simulink model "bldc_control"  (R2014b)
settings: Solver=ode3  StartTime=0.0  StopTime=tdur  FixedStep=dt  RelTol=1e-3
values from neighbouring files (symbols this model uses):
  CTRL_MODE = 1    [bldc_control_run.m]
  dt = 0.2    [bldc_control_run.m]    (also in bldc_discrete.m = CONST.dt; bldc_discrete_model.m = CONST.dt; bldc_discrete_torque.m = CONST.dt; bldc_speed_discrete.m = CONST.dt)
  i_kd = 0    [bldc_control_run.m]
  i_ki = 1e3    (= 1000)    [bldc_control_run.m]
  i_kp = 10    [bldc_control_run.m]
  i_tgt = 0.15    [bldc_control_run.m]
  J = 978.548e-6    (= 0.000978548)    [bldc_control_run.m]    (also in bldc_discrete.m = CONST.J; bldc_discrete_model.m = CONST.J; bldc_motor.m = CONST.J; bldc_speed.m = CONST.J)
  spd_kd = 0.00    (= 0)    [bldc_control_run.m]    (also in bldc_speed_discrete.m = CONST.spd_kd)
  spd_ki = 0.10    (= 0.1)    [bldc_control_run.m]    (also in bldc_speed_discrete.m = CONST.spd_ki)
  spd_kp = 0.50    (= 0.5)    [bldc_control_run.m]    (also in bldc_speed_discrete.m = CONST.spd_kp)
  theta_m_0 = 0    [bldc_control_run.m]
  thold = 0.5    [bldc_control_run.m]
  trq_kd = 0    [bldc_control_run.m]    (also in bldc_discrete_torque.m = CONST.trq_kd)
  trq_ki = 5e4    (= 50000)    [bldc_control_run.m]    (also in bldc_discrete_torque.m = CONST.trq_ki)
  trq_kp = 1e3    (= 1000)    [bldc_control_run.m]    (also in bldc_discrete_torque.m = CONST.trq_kp)
  trq_tgt = 0.1e-3    (= 0.0001)    [bldc_control_run.m]
  V_tgt = 2.1    [bldc_control_run.m]
  Vmax = 24    [bldc_control_run.m]
  w_m_0 = 0    [bldc_control_run.m]
  w_tgt = rpm2rps(2000)    [bldc_control_run.m]
libraries: simulink x1, tool x1
settings Model: Creator=root  LastModifiedBy=root
settings DebuggingCC: FrameProcessingCompatibilityMsg=error

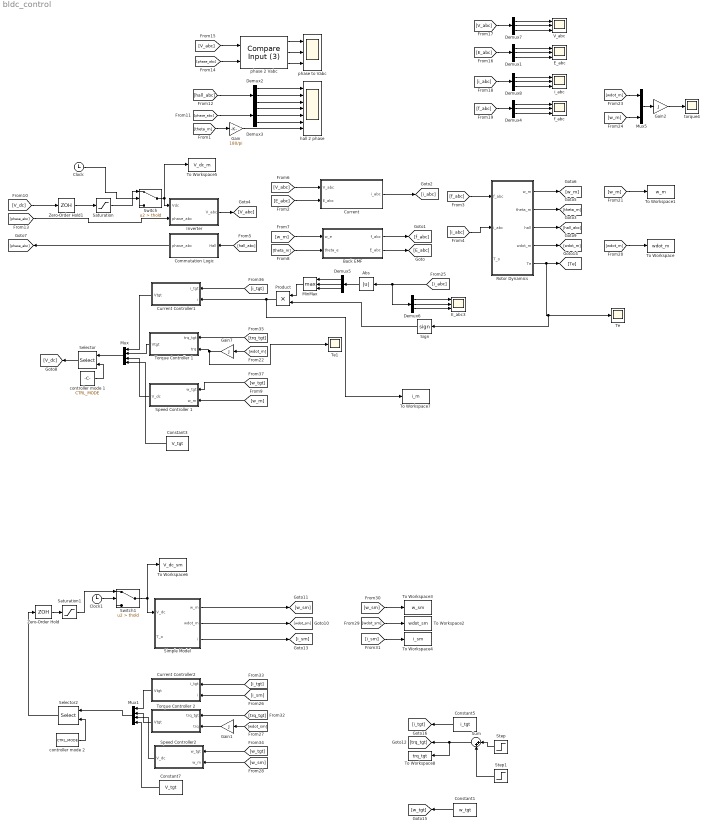
== system bldc_control ==
  Abs : Abs
  Back EMF : Subsystem
  Clock : Clock
  Clock1 : Clock
  Commutation Logic : Subsystem
  Constant1 : Constant  Value=w_tgt
  Constant3 : Constant  Value=V_tgt
  Constant5 : Constant  Value=i_tgt
  Constant7 : Constant  Value=V_tgt
  Current : Subsystem
  Current Controller1 : Subsystem
  Current Controller2 : Subsystem
  Demux{1..8} (8 alike) : Demux  Outputs=3
  E_abc : Scope  NumInputPorts=3
      settings: TimeRange=60  YMin=18000~-5~-5  YMax=20500~5~5  SaveName=ScopeData6
  E_abc3 : Scope  NumInputPorts=3
      settings: TimeRange=5  YMin=-0.05~-0.05~-0.05  YMax=0.05~0.05~0.05  SaveName=ScopeData3
  Gain : Gain  Gain=180/pi
  Gain1 : Gain  Gain=J
  Gain2 : Gain  Gain=J
  Gain7 : Gain  Gain=J
  Inverter : Subsystem
  MinMax : MinMax  Function=max  Inputs=3
  Mux : Mux
  Mux1 : Mux
  Mux5 : Mux  Inputs=3
  Product : Product
  Rotor Dynamics : Subsystem
  Saturation : Saturate  UpperLimit=Vmax  LowerLimit=-Vmax
  Saturation1 : Saturate  UpperLimit=Vmax  LowerLimit=-Vmax
  Selector : Selector  InputPortWidth=4  IndexOptions=Starting index (port)
  Selector2 : Selector  InputPortWidth=4  IndexOptions=Starting index (port)
  Sign : Signum
  Simple Model : Subsystem
  Speed Controller 1 : Subsystem
  Speed Controller2 : Subsystem
  Step : Step  Time=0  After=trq_tgt  SampleTime=0
  Step1 : Step  Time=5  After=-2*trq_tgt  SampleTime=0
  Sum : Sum  Inputs=|++
  Switch : Switch  Criteria=u2 > Threshold  Threshold=thold
  Switch1 : Switch  Criteria=u2 > Threshold  Threshold=thold
  Te : Scope
      settings: TimeRange=1  YMin=1.2e-05  YMax=2.4e-05  SaveName=ScopeData7
  Te1 : Scope
      settings: TimeRange=1  YMin=1.2e-05  YMax=2.4e-05
  To Workspace : ToWorkspace  VariableName=wdot_m  SampleTime=-1
  To Workspace1 : ToWorkspace  VariableName=w_m  SampleTime=-1
  To Workspace2 : ToWorkspace  VariableName=wdot_sm  SampleTime=-1
  To Workspace3 : ToWorkspace  VariableName=w_sm  SampleTime=-1
  To Workspace4 : ToWorkspace  VariableName=i_sm  SampleTime=-1
  To Workspace5 : ToWorkspace  VariableName=V_dc_m  SampleTime=-1
  To Workspace6 : ToWorkspace  VariableName=V_dc_sm  SampleTime=-1
  To Workspace7 : ToWorkspace  VariableName=i_m  SampleTime=-1
  To Workspace8 : ToWorkspace  VariableName=trq_tgt  SampleTime=-1
  Torque Controller 1 : Subsystem
  Torque Controller 2 : Subsystem
  V_abc : Scope  NumInputPorts=3
      settings: TimeRange=60  YMin=18000~-5~-5  YMax=20500~5~5  SaveName=ScopeData5
  Zero-Order Hold : ZeroOrderHold  SampleTime=dt
  Zero-Order Hold1 : ZeroOrderHold  SampleTime=dt
  controller mode 1 : Constant  Value=CTRL_MODE
  controller mode 2 : Constant  Value=CTRL_MODE
  f_abc : Scope  NumInputPorts=3
      settings: TimeRange=60  YMin=18000~-5~-5  YMax=20500~5~5
  hall 2 phase : Scope  NumInputPorts=7
      settings: TimeRange=5  YMin=0~0~0~-1~-1~-1~-200  YMax=1~1~1~1~1~1~200  SaveName=ScopeData8
  i_abc : Scope  NumInputPorts=3
      settings: TimeRange=60  YMin=18000~-5~-5  YMax=20500~5~5  SaveName=ScopeData4
  phase 2 Vabc : tool/Compare Input (3)
  phase to Vabc : Scope  NumInputPorts=3
      settings: TimeRange=5  YMin=-1~-1~-1  YMax=1~1~1  SaveName=ScopeData2
  torque4 : Scope
      settings: TimeRange=1  YMin=1.2e-05  YMax=2.4e-05  SaveName=ScopeData11
  wires:
  [E_abc] -> Current/2(E_abc)
  Back EMF/2(E_abc) -> [E_abc]
  Back EMF/1(f_abc) -> [f_abc]
  [i_abc] -> Rotor Dynamics/2(i_abc)
  Rotor Dynamics/3(hall) -> [hall_abc]
  Commutation Logic/1(phase_abc) -> [phase_abc]
  [V_abc] -> Current/1(V_abc)
  Rotor Dynamics/2(theta_m) -> [theta_m]
  Rotor Dynamics/1(w_m) -> [w_m]
  [theta_m] -> Back EMF/2(theta_e)
  [w_m] -> Back EMF/1(w_e)
  Inverter/1(V_abc) -> [V_abc]
  [hall_abc] -> Commutation Logic/1("Hall ")
  Rotor Dynamics/4(wdot_m) -> [wdot_m]
  Simple Model/1(w_m) -> [w_sm]
  Demux1/3 -> E_abc/3
  Demux1/2 -> E_abc/2
  Demux1/1 -> E_abc/1
  Demux4/3 -> f_abc/3
  Demux4/2 -> f_abc/2
  Demux4/1 -> f_abc/1
  [f_abc] -> Rotor Dynamics/1(f_abc)
  phase 2 Vabc/3 -> phase to Vabc/3
  phase 2 Vabc/2 -> phase to Vabc/2
  phase 2 Vabc/1 -> phase to Vabc/1
  Demux5/1 -> MinMax/1
  Demux5/3 -> MinMax/3
  Demux5/2 -> MinMax/2
  [V_dc] -> Zero-Order Hold1/1
  Current/1(i_abc) -> [i_abc]
  Abs/1 -> Demux5/1
  Simple Model/3(i) -> [i_sm]
  Demux6/3 -> E_abc3/3
  Demux6/2 -> E_abc3/2
  Demux6/1 -> E_abc3/1
  Simple Model/2(wdot_m) -> [wdot_sm]
  Mux5/1 -> Gain2/1
  Constant5/1 -> [i_tgt]
  [i_tgt] -> Current Controller1/1(i_tgt)
  MinMax/1 -> Product/1
  Demux2/3 -> hall 2 phase/3
  Demux2/2 -> hall 2 phase/2
  Demux2/1 -> hall 2 phase/1
  Demux3/2 -> hall 2 phase/5
  Demux3/1 -> hall 2 phase/4
  Demux3/3 -> hall 2 phase/6
  [theta_m] -> Gain/1
  [phase_abc] -> Demux3/1
  Gain/1 -> hall 2 phase/7
  [hall_abc] -> Demux2/1
  [phase_abc] -> Inverter/2(phase_abc)
  [phase_abc] -> phase 2 Vabc/2
  [V_abc] -> phase 2 Vabc/1
  [E_abc] -> Demux1/1
  Demux7/3 -> V_abc/3
  Demux7/2 -> V_abc/2
  Demux7/1 -> V_abc/1
  [V_abc] -> Demux7/1
  Saturation/1 -> Switch/1
  Saturation1/1 -> Switch1/1
  Mux/1 -> Selector/1
  Demux8/3 -> i_abc/3
  Demux8/2 -> i_abc/2
  Demux8/1 -> i_abc/1
  [i_abc] -> Demux8/1
  [f_abc] -> Demux4/1
  [wdot_m] -> To Workspace/1
  [w_m] -> To Workspace1/1
  Gain7/1 -> Te1/1, Torque Controller 1/2(trq)
  [wdot_m] -> Gain7/1
  [wdot_m] -> Mux5/1
  [w_m] -> Mux5/3
  Gain2/1 -> torque4/1
  [i_abc] -> Demux6/1, Abs/1
  [i_sm] -> Current Controller2/2(i)
  [w_sm] -> Speed Controller2/2(w_m)
  [wdot_sm] -> Gain1/1
  Gain1/1 -> Torque Controller 2/2(trq)
  [w_tgt] -> Speed Controller 1/1(w_tgt)
  [w_m] -> Speed Controller 1/2(w_m)
  Rotor Dynamics/5(Te) -> Sign/1, Te/1, [Te]
  Current Controller1/1(Vtgt) -> Mux/1
  Torque Controller 1/1(Vtgt) -> Mux/2
  Speed Controller 1/1(V_dc) -> Mux/3
  Selector/1 -> [V_dc]
  Sign/1 -> Product/2
  Mux1/1 -> Selector2/1
  Selector2/1 -> Zero-Order Hold/1
  Current Controller2/1(Vtgt) -> Mux1/1
  Torque Controller 2/1(Vtgt) -> Mux1/2
  Speed Controller2/1(V_dc) -> Mux1/3
  [wdot_sm] -> To Workspace2/1
  [w_sm] -> To Workspace3/1
  [i_sm] -> To Workspace4/1
  controller mode 1/1 -> Selector/2
  controller mode 2/1 -> Selector2/2
  [trq_tgt] -> Torque Controller 1/1(trq_tgt)
  Product/1 -> Current Controller1/2(i), To Workspace7/1
  Constant3/1 -> Mux/4
  Constant7/1 -> Mux1/4
  Clock/1 -> Switch/2
  Switch/1 -> Inverter/1(Vdc), To Workspace5/1
  Clock1/1 -> Switch1/2
  Switch1/1 -> Simple Model/1(V_dc), To Workspace6/1
  Zero-Order Hold/1 -> Saturation1/1
  Zero-Order Hold1/1 -> Saturation/1
  Sum/1 -> [trq_tgt], To Workspace8/1
  [trq_tgt] -> Torque Controller 2/1(trq_tgt)
  [i_tgt] -> Current Controller2/1(i_tgt)
  [w_tgt] -> Speed Controller2/1(w_tgt)
  Constant1/1 -> [w_tgt]
  Step/1 -> Sum/1
  Step1/1 -> Sum/2

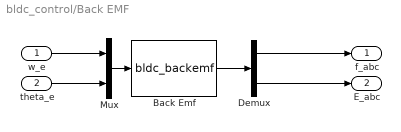
== system bldc_control/Back EMF ==
  w_e : Inport
  theta_e : Inport  Port=2
  Back Emf : MATLABFcn  MATLABFcn=bldc_backemf  OutputDimensions=[6,1]  Output1D=off
  Demux : Demux  Outputs=[3 3]
  Mux : Mux  Inputs=[1;1]
  f_abc : Outport
  E_abc : Outport  Port=2
  wires:
  Demux/2 -> E_abc/1
  Demux/1 -> f_abc/1
  w_e/1 -> Mux/1
  Back Emf/1 -> Demux/1
  Mux/1 -> Back Emf/1
  theta_e/1 -> Mux/2

== system bldc_control/Commutation Logic ==
  "Hall " : Inport
  bldc_commutation : MATLABFcn  MATLABFcn=bldc_commutation  OutputDimensions=[3,1]  Output1D=off
  phase_abc : Outport
  wires:
  "Hall "/1 -> bldc_commutation/1
  bldc_commutation/1 -> phase_abc/1

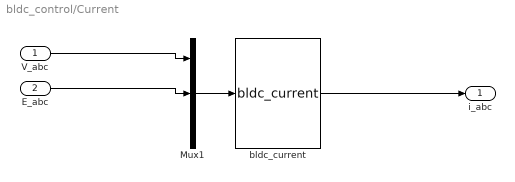
== system bldc_control/Current ==
  V_abc : Inport
  E_abc : Inport  Port=2
  Mux1 : Mux  Inputs=[3;3;3]
  bldc_current : MATLABFcn  MATLABFcn=bldc_current  OutputDimensions=[3,1]  Output1D=off
  i_abc : Outport
  wires:
  Mux1/1 -> bldc_current/1
  E_abc/1 -> Mux1/2
  V_abc/1 -> Mux1/1
  bldc_current/1 -> i_abc/1

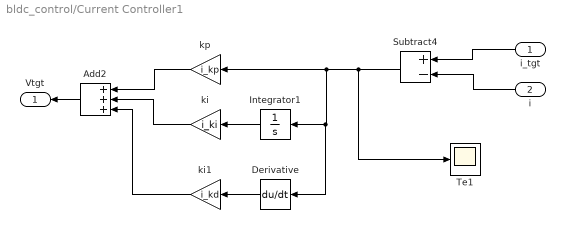
== system bldc_control/Current Controller1 ==
  i_tgt : Inport
  i : Inport  Port=2
  Add2 : Sum  Inputs=+++
  Derivative : Derivative
  Integrator1 : Integrator
  Subtract4 : Sum  Inputs=+-
  Te1 : Scope
      settings: TimeRange=1  YMin=1.2e-05  YMax=2.4e-05  SaveName=ScopeData10
  ki : Gain  Gain=i_ki
  ki1 : Gain  Gain=i_kd
  kp : Gain  Gain=i_kp
  Vtgt : Outport
  wires:
  i_tgt/1 -> Subtract4/1
  i/1 -> Subtract4/2
  Integrator1/1 -> ki/1
  Add2/1 -> Vtgt/1
  kp/1 -> Add2/1
  ki/1 -> Add2/2
  Derivative/1 -> ki1/1
  ki1/1 -> Add2/3
  Subtract4/1 -> Te1/1, kp/1, Derivative/1, Integrator1/1

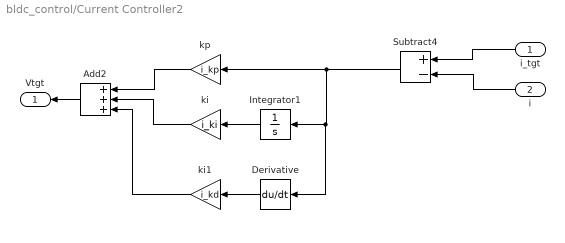
== system bldc_control/Current Controller2 ==
  i_tgt : Inport
  i : Inport  Port=2
  Add2 : Sum  Inputs=+++
  Derivative : Derivative
  Integrator1 : Integrator
  Subtract4 : Sum  Inputs=+-
  ki : Gain  Gain=i_ki
  ki1 : Gain  Gain=i_kd
  kp : Gain  Gain=i_kp
  Vtgt : Outport
  wires:
  i_tgt/1 -> Subtract4/1
  i/1 -> Subtract4/2
  Integrator1/1 -> ki/1
  Subtract4/1 -> kp/1, Derivative/1, Integrator1/1
  Add2/1 -> Vtgt/1
  kp/1 -> Add2/1
  ki/1 -> Add2/2
  Derivative/1 -> ki1/1
  ki1/1 -> Add2/3

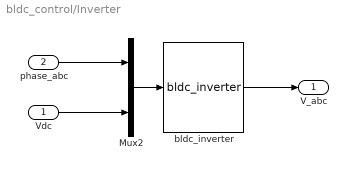
== system bldc_control/Inverter ==
  Vdc : Inport
  phase_abc : Inport  Port=2
  Mux2 : Mux  Inputs=[3;1]
  bldc_inverter : MATLABFcn  MATLABFcn=bldc_inverter  OutputDimensions=[3,1]  Output1D=off
  V_abc : Outport
  wires:
  phase_abc/1 -> Mux2/1
  Vdc/1 -> Mux2/2
  Mux2/1 -> bldc_inverter/1
  bldc_inverter/1 -> V_abc/1

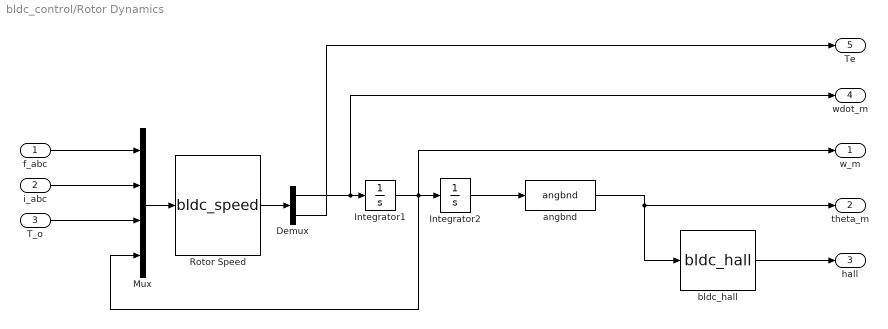
== system bldc_control/Rotor Dynamics ==
  f_abc : Inport
  i_abc : Inport  Port=2
  T_o : Inport  Port=3
  Demux : Demux  Outputs=2
  Integrator1 : Integrator  InitialCondition=w_m_0
  Integrator2 : Integrator  InitialCondition=theta_m_0
  Mux : Mux  Inputs=[3;3;1;1]
  Rotor Speed : MATLABFcn  MATLABFcn=bldc_speed  OutputDimensions=[2,1]  Output1D=off
  angbnd : MATLABFcn  MATLABFcn=angbnd
  bldc_hall : MATLABFcn  MATLABFcn=bldc_hall  Output1D=off
  w_m : Outport
  theta_m : Outport  Port=2
  hall : Outport  Port=3
  wdot_m : Outport  Port=4
  Te : Outport  Port=5
  wires:
  Rotor Speed/1 -> Demux/1
  T_o/1 -> Mux/3
  i_abc/1 -> Mux/2
  Mux/1 -> Rotor Speed/1
  f_abc/1 -> Mux/1
  bldc_hall/1 -> hall/1
  Integrator2/1 -> angbnd/1
  Integrator1/1 -> w_m/1, Mux/4, Integrator2/1
  angbnd/1 -> theta_m/1, bldc_hall/1
  Demux/1 -> wdot_m/1, Integrator1/1
  Demux/2 -> Te/1

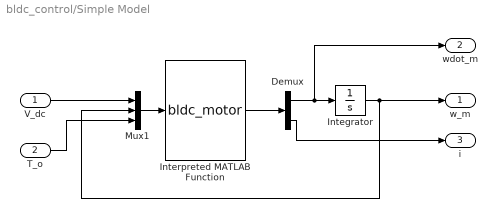
== system bldc_control/Simple Model ==
  V_dc : Inport
  T_o : Inport  Port=2
  Demux : Demux  Outputs=2
  Integrator : Integrator  InitialCondition=w_m_0
  Interpreted MATLAB Function : MATLABFcn  MATLABFcn=bldc_motor  OutputDimensions=[2,1]  Output1D=off
  Mux1 : Mux  Inputs=3
  w_m : Outport
  wdot_m : Outport  Port=2
  i : Outport  Port=3
  wires:
  V_dc/1 -> Mux1/1
  Mux1/1 -> Interpreted MATLAB Function/1
  Integrator/1 -> Mux1/2, w_m/1
  Interpreted MATLAB Function/1 -> Demux/1
  Demux/1 -> Integrator/1, wdot_m/1
  Demux/2 -> i/1
  T_o/1 -> Mux1/3

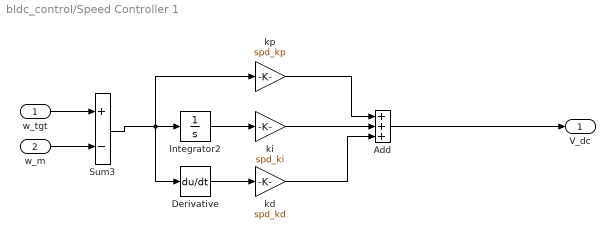
== system bldc_control/Speed Controller 1 ==
  w_tgt : Inport
  w_m : Inport  Port=2
  Add : Sum  Inputs=+++
  Derivative : Derivative
  Integrator2 : Integrator
  Sum3 : Sum  Inputs=+-
  kd : Gain  Gain=spd_kd
  ki : Gain  Gain=spd_ki
  kp : Gain  Gain=spd_kp
  V_dc : Outport
  wires:
  Add/1 -> V_dc/1
  Integrator2/1 -> ki/1
  Sum3/1 -> Derivative/1, Integrator2/1, kp/1
  Derivative/1 -> kd/1
  kp/1 -> Add/1
  w_tgt/1 -> Sum3/1
  w_m/1 -> Sum3/2
  ki/1 -> Add/2
  kd/1 -> Add/3

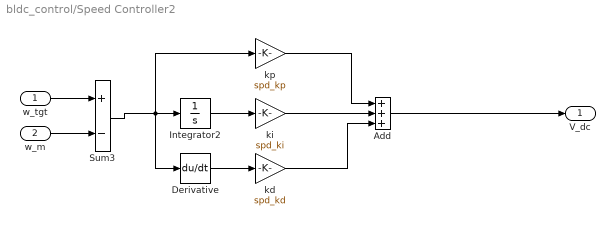
== system bldc_control/Speed Controller2 ==
  w_tgt : Inport
  w_m : Inport  Port=2
  Add : Sum  Inputs=+++
  Derivative : Derivative
  Integrator2 : Integrator
  Sum3 : Sum  Inputs=+-
  kd : Gain  Gain=spd_kd
  ki : Gain  Gain=spd_ki
  kp : Gain  Gain=spd_kp
  V_dc : Outport
  wires:
  Integrator2/1 -> ki/1
  Sum3/1 -> Derivative/1, Integrator2/1, kp/1
  Derivative/1 -> kd/1
  kp/1 -> Add/1
  Add/1 -> V_dc/1
  w_tgt/1 -> Sum3/1
  w_m/1 -> Sum3/2
  ki/1 -> Add/2
  kd/1 -> Add/3

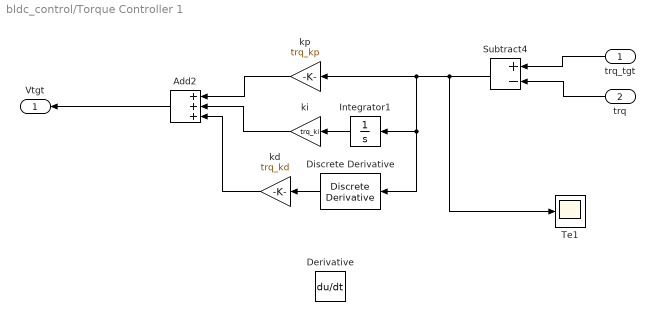
== system bldc_control/Torque Controller 1 ==
  trq_tgt : Inport
  trq : Inport  Port=2
  Add2 : Sum  Inputs=+++
  Derivative : Derivative
  Discrete Derivative : simulink/Discrete/Discrete Derivative  gainval=1.0  ICPrevScaledInput=0.0  InputProcessing=Inherited  OutMin=[]  OutMax=[]  OutDataType=fixdt(1, 16)  OutScaling=2^-10  DoSatur=off
  Integrator1 : Integrator
  Subtract4 : Sum  Inputs=+-
  Te1 : Scope
      settings: TimeRange=1  YMin=1.2e-05  YMax=2.4e-05  SaveName=ScopeData9
  kd : Gain  Gain=trq_kd
  ki : Gain  Gain=trq_ki
  kp : Gain  Gain=trq_kp
  Vtgt : Outport
  wires:
  trq_tgt/1 -> Subtract4/1
  trq/1 -> Subtract4/2
  Integrator1/1 -> ki/1
  Add2/1 -> Vtgt/1
  kp/1 -> Add2/1
  ki/1 -> Add2/2
  Discrete Derivative/1 -> kd/1
  kd/1 -> Add2/3
  Subtract4/1 -> Te1/1, kp/1, Discrete Derivative/1, Integrator1/1

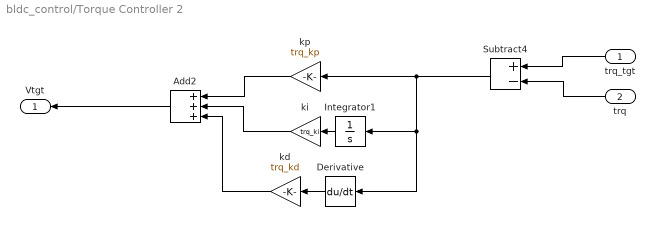
== system bldc_control/Torque Controller 2 ==
  trq_tgt : Inport
  trq : Inport  Port=2
  Add2 : Sum  Inputs=+++
  Derivative : Derivative
  Integrator1 : Integrator
  Subtract4 : Sum  Inputs=+-
  kd : Gain  Gain=trq_kd
  ki : Gain  Gain=trq_ki
  kp : Gain  Gain=trq_kp
  Vtgt : Outport
  wires:
  trq_tgt/1 -> Subtract4/1
  trq/1 -> Subtract4/2
  Integrator1/1 -> ki/1
  Add2/1 -> Vtgt/1
  kp/1 -> Add2/1
  ki/1 -> Add2/2
  Derivative/1 -> kd/1
  kd/1 -> Add2/3
  Subtract4/1 -> kp/1, Derivative/1, Integrator1/1
